simulink model "de2theta"  (R2020b)
settings: Solver=VariableStepAuto  StartTime=0.0  StopTime=20.0  RelTol=1e-3
undefined symbols (not defined in the file or in its folder): den_sp, num_sp
libraries: simulink_extras x3
settings Model: Creator=JaimeParker  LastModifiedBy=JaimeParker

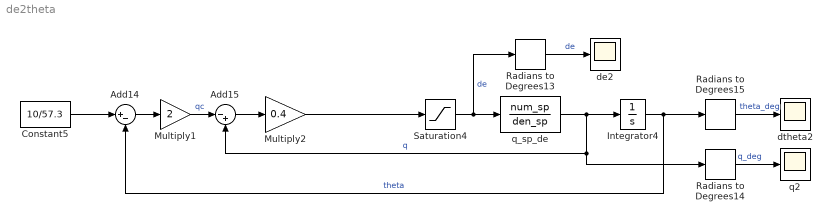
== system de2theta ==
  Add14 : Sum  Inputs=|+-
  Add15 : Sum  Inputs=|-+
  Constant5 : Constant  Value=10/57.3
  Integrator4 : Integrator
  Multiply1 : Gain  Gain=2
  Multiply2 : Gain  Gain=0.4
  Radians to Degrees13 : simulink_extras/Transformations/Radians to Degrees
  Radians to Degrees14 : simulink_extras/Transformations/Radians to Degrees
  Radians to Degrees15 : simulink_extras/Transformations/Radians to Degrees
  Saturation4 : Saturate  UpperLimit=20/57.3  LowerLimit=-20/57.3
  de2 : Scope
  dtheta2 : Scope
  q2 : Scope
  q_sp_de : TransferFcn  Numerator=num_sp  Denominator=den_sp
  wires:
  Radians to Degrees14/1 -> q2/1  "q_deg"
  Multiply2/1 -> Saturation4/1
  Multiply1/1 -> Add15/1  "qc"
  Radians to Degrees15/1 -> dtheta2/1  "theta_deg"
  Saturation4/1 -> q_sp_de/1, Radians to Degrees13/1  "de"
  Radians to Degrees13/1 -> de2/1  "de"
  Integrator4/1 -> Radians to Degrees15/1, Add14/2  "theta"
  Add15/1 -> Multiply2/1
  q_sp_de/1 -> Integrator4/1, Add15/2, Radians to Degrees14/1  "q"
  Add14/1 -> Multiply1/1
  Constant5/1 -> Add14/1
